simulink model "Traffic_controller_2"  (R2024b)
settings: Solver=VariableStepAuto  StartTime=0.0  StopTime=10.0  RelTol=1e-3
(part 2 of 2)

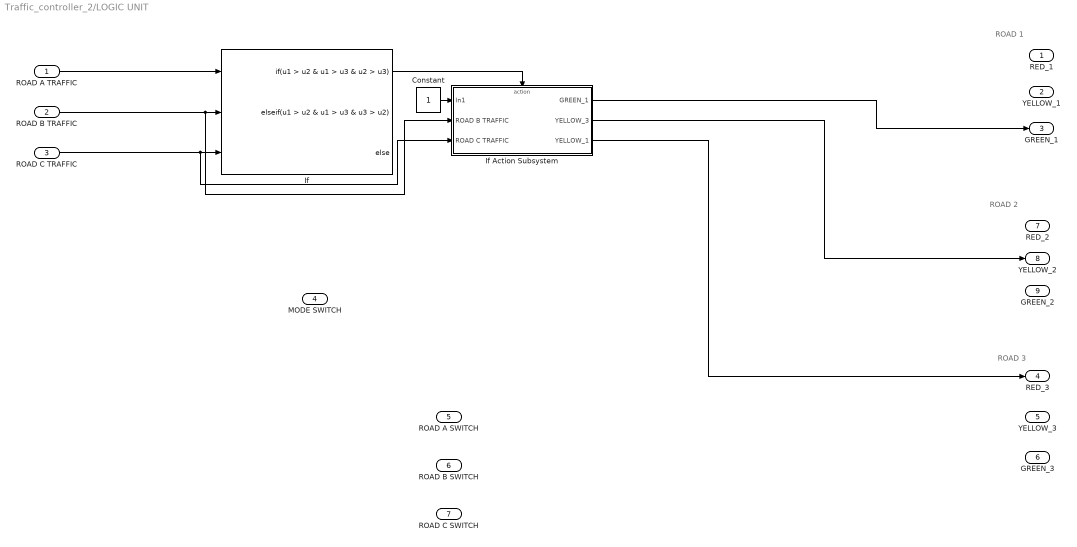
== system Traffic_controller_2/LOGIC UNIT ==
  note: ROAD 2
  note: ROAD 3
  note: ROAD 1
  ROAD A TRAFFIC : Inport
  ROAD B TRAFFIC : Inport  Port=2
  ROAD C TRAFFIC : Inport  Port=3
  MODE SWITCH : Inport  Port=4
  ROAD A SWITCH : Inport  Port=5
  ROAD B SWITCH : Inport  Port=6
  ROAD C SWITCH : Inport  Port=7
  Constant : Constant
  If : If  NumInputs=3  IfExpression=u1 > u2 & u1 > u3 & u2 > u3  ElseIfExpressions=u1 > u2 & u1 > u3 & u3 > u2
  If Action Subsystem : Subsystem  TreatAsAtomicUnit=on
  RED_1 : Outport
  YELLOW_1 : Outport  Port=2
  GREEN_1 : Outport  Port=3
  RED_3 : Outport  Port=4
  YELLOW_3 : Outport  Port=5
  GREEN_3 : Outport  Port=6
  RED_2 : Outport  Port=7
  YELLOW_2 : Outport  Port=8
  GREEN_2 : Outport  Port=9
  wires:
  ROAD B TRAFFIC/1 -> If Action Subsystem/2(ROAD B TRAFFIC), If/2
  ROAD A TRAFFIC/1 -> If/1
  ROAD C TRAFFIC/1 -> If Action Subsystem/3(ROAD C TRAFFIC), If/3
  Constant/1 -> If Action Subsystem/1(In1)
  If/1 -> If Action Subsystem/Action
  If Action Subsystem/1(GREEN_1) -> GREEN_1/1
  If Action Subsystem/2(YELLOW_3) -> YELLOW_2/1
  If Action Subsystem/3(YELLOW_1) -> RED_3/1

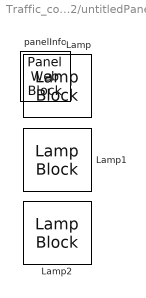
== system Traffic_controller_2/untitledPanel ==
  Lamp : LampBlock  Tag=HiddenForWebPanel  PanelInfo="{\"height\":63,\"left\":18,\"panelId\":\"panelId-7e957e8d-dff8-4cec-a468-1be17fa4fdbd\",\"top\":18,\"type\":\"panelChild\",\"version\":\"2019b\",\"width\":68,\"zIndex\":1500004}"  LabelPosition=Hide
  Lamp1 : LampBlock  Tag=HiddenForWebPanel  PanelInfo="{\"height\":63,\"left\":18,\"panelId\":\"panelId-7e957e8d-dff8-4cec-a468-1be17fa4fdbd\",\"top\":92,\"type\":\"panelChild\",\"version\":\"2019b\",\"width\":68,\"zIndex\":1500002}"  LabelPosition=Hide
  Lamp2 : LampBlock  Tag=HiddenForWebPanel  PanelInfo="{\"height\":63,\"left\":18,\"panelId\":\"panelId-7e957e8d-dff8-4cec-a468-1be17fa4fdbd\",\"top\":165,\"type\":\"panelChild\",\"version\":\"2019b\",\"width\":68,\"zIndex\":1500006}"  LabelPosition=Hide
  panelInfo : PanelWebBlock  Tag=HiddenForWebPanel  PanelInfo="{\"compacted\":false,\"height\":250,\"isActiveTab\":true,\"left\":1468,\"name\":\"Panel\",\"panelId\":\"panelId-7e957e8d-dff8-4cec-a468-1be17fa4fdbd\",\"tabIndex\":0,\"tabbedSetId\":\"tabbedSet9836852289\",\"top\":0,\"type\":\"panel\",\"version\":\"2019b\",\"visible\":true,\"width\":108,\"zIndex\":1500002}"

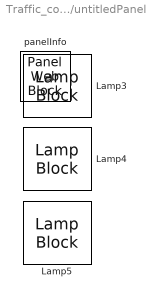
== system Traffic_controller_2/untitledPanel1 ==
  Lamp3 : LampBlock  Tag=HiddenForWebPanel  PanelInfo="{\"height\":63,\"left\":18,\"panelId\":\"panelId-c0389c40-72cf-4991-ab23-55a45b104da0\",\"top\":18,\"type\":\"panelChild\",\"version\":\"2019b\",\"width\":68,\"zIndex\":1500006}"  LabelPosition=Hide
  Lamp4 : LampBlock  Tag=HiddenForWebPanel  PanelInfo="{\"height\":63,\"left\":18,\"panelId\":\"panelId-c0389c40-72cf-4991-ab23-55a45b104da0\",\"top\":91,\"type\":\"panelChild\",\"version\":\"2019b\",\"width\":68,\"zIndex\":1500002}"  LabelPosition=Hide
  Lamp5 : LampBlock  Tag=HiddenForWebPanel  PanelInfo="{\"height\":63,\"left\":18,\"panelId\":\"panelId-c0389c40-72cf-4991-ab23-55a45b104da0\",\"top\":165,\"type\":\"panelChild\",\"version\":\"2019b\",\"width\":68,\"zIndex\":1500004}"  LabelPosition=Hide
  panelInfo : PanelWebBlock  Tag=HiddenForWebPanel  PanelInfo="{\"compacted\":false,\"height\":250,\"isActiveTab\":true,\"left\":1475,\"name\":\"Panel1\",\"panelId\":\"panelId-c0389c40-72cf-4991-ab23-55a45b104da0\",\"tabIndex\":0,\"tabbedSetId\":\"tabbedSet4509576382\",\"top\":457,\"type\":\"panel\",\"version\":\"2019b\",\"visible\":true,\"width\":108,\"zIndex\":1500004}"

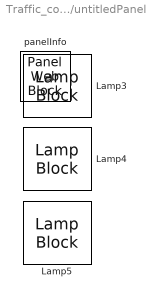
== system Traffic_controller_2/untitledPanel2 ==
  Lamp3 : LampBlock  Tag=HiddenForWebPanel  PanelInfo="{\"height\":63,\"left\":18,\"panelId\":\"panelId-715a9372-3f55-44a8-94da-ec86e91b5bde\",\"top\":18,\"type\":\"panelChild\",\"version\":\"2019b\",\"width\":68,\"zIndex\":1500006}"  LabelPosition=Hide
  Lamp4 : LampBlock  Tag=HiddenForWebPanel  PanelInfo="{\"height\":63,\"left\":18,\"panelId\":\"panelId-715a9372-3f55-44a8-94da-ec86e91b5bde\",\"top\":91,\"type\":\"panelChild\",\"version\":\"2019b\",\"width\":68,\"zIndex\":1500002}"  LabelPosition=Hide
  Lamp5 : LampBlock  Tag=HiddenForWebPanel  PanelInfo="{\"height\":63,\"left\":18,\"panelId\":\"panelId-715a9372-3f55-44a8-94da-ec86e91b5bde\",\"top\":165,\"type\":\"panelChild\",\"version\":\"2019b\",\"width\":68,\"zIndex\":1500004}"  LabelPosition=Hide
  panelInfo : PanelWebBlock  Tag=HiddenForWebPanel  PanelInfo="{\"compacted\":false,\"height\":250,\"isActiveTab\":true,\"left\":1341,\"name\":\"Panel2\",\"panelId\":\"panelId-715a9372-3f55-44a8-94da-ec86e91b5bde\",\"tabIndex\":0,\"tabbedSetId\":\"tabbedSet1869882240\",\"top\":238,\"type\":\"panel\",\"version\":\"2019b\",\"visible\":true,\"width\":108,\"zIndex\":1500006}"

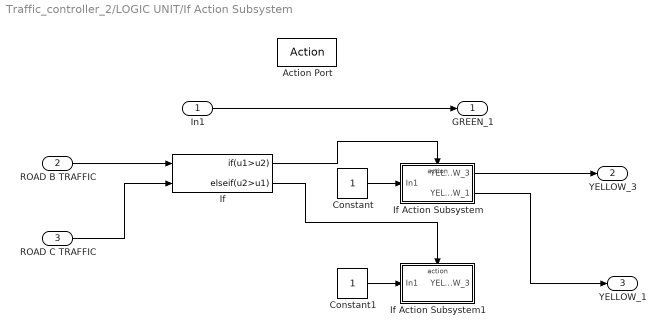
== system Traffic_controller_2/LOGIC UNIT/If Action Subsystem ==
  In1 : Inport
  ROAD B TRAFFIC : Inport  Port=2
  ROAD C TRAFFIC : Inport  Port=3
  Action Port : ActionPort  ActionPortLabel=if(u1 > u2 & u1 > u3 & u2 > u3)
  Constant : Constant
  Constant1 : Constant
  If : If  NumInputs=2  IfExpression=u1>u2  ElseIfExpressions=u2>u1  ShowElse=off
  If Action Subsystem : Subsystem  TreatAsAtomicUnit=on
  If Action Subsystem1 : Subsystem  TreatAsAtomicUnit=on
  GREEN_1 : Outport
  YELLOW_3 : Outport  Port=2
  YELLOW_1 : Outport  Port=3
  wires:
  In1/1 -> GREEN_1/1
  ROAD B TRAFFIC/1 -> If/1
  ROAD C TRAFFIC/1 -> If/2
  Constant/1 -> If Action Subsystem/1(In1)
  If/1 -> If Action Subsystem/Action
  Constant1/1 -> If Action Subsystem1/1(In1)
  If/2 -> If Action Subsystem1/Action
  If Action Subsystem/1(YELLOW_3) -> YELLOW_3/1
  If Action Subsystem/2(YELLOW_1) -> YELLOW_1/1

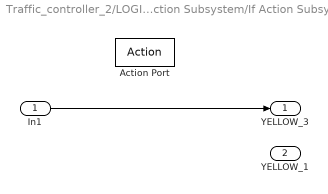
== system Traffic_controller_2/LOGIC UNIT/If Action Subsystem/If Action Subsystem ==
  In1 : Inport
  Action Port : ActionPort  ActionPortLabel=if(u1>u2)
  YELLOW_3 : Outport
  YELLOW_1 : Outport  Port=2
  wires:
  In1/1 -> YELLOW_3/1

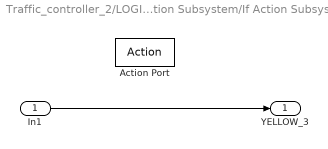
== system Traffic_controller_2/LOGIC UNIT/If Action Subsystem/If Action Subsystem1 ==
  In1 : Inport
  Action Port : ActionPort  ActionPortLabel=elseif(u2>u1)
  YELLOW_3 : Outport
  wires:
  In1/1 -> YELLOW_3/1
